simulink model "ctrl_student_HIL"  (R2015a)
settings: Solver=ode3  StartTime=0.0  StopTime=inf  FixedStep=0.01  RelTol=1e-3
undefined symbols (not defined in the file): DesiredPath, Elipscenter_radi, eta_dot_ini, K, K1, K2, l1, l2, l3, LAW, lim, lim_2, m, mu, pd, T_initialDP, U_ref
libraries: simulink x1
(part 4 of 4)

== matlab function ctrl_student_HIL/ControllerAndParanetrization/Controller1/Controller/Controller/MATLAB Function ==
  data: u input; D output; v input; r input
function D = fcn(u,v,r)
%% Damping coefficients
% Comments at the end of the lines indicate the old values used.
X_u		= -0.6555;		X_v		= 0;
X_uu 	= 0.3545;		X_vv	= -2.443;
X_uuu 	= -3.787;		X_vvv	= 0;

Y_v		= -1.33; 			Y_r		= -7.250; % Y_r
Y_vv	= -2.776;			Y_rr	= -3.450; % Y_rr
Y_vvv	= -64.91;			Y_rrr	= 0;
						
Y_rv	= -0.805;			Y_vr	= -0.845; % Y_rv, Y_vr

N_v		= 0;				N_r		= -1.900; % N_r
N_vv	= -0.2088;			N_rr	= -0.750; % N_rr
N_vvv	= 0;				N_rrr	= 0;
N_rv	= 0.130;			N_vr	= 0.080; % N_rv, N_vr
d_11 = -X_u - X_uu*u - X_uuu*u^2;
d_22 = -Y_v - Y_vv*v - Y_vvv*v^2 - Y_rv*abs(r);
d_33 = -N_r - N_rr*abs(r) - N_rrr*r^2 - N_vr*abs(v); % using abs(r)

d_12 = -X_v - X_vv*v - X_vvv*v^2;
d_23 = -Y_r - Y_rr*abs(r) - Y_rrr*r^2 - Y_vr*abs(v);
d_32 = -N_v - N_vv*v - N_vvv*v^2 - N_rv*abs(r);

D    = [d_11 0    0
        0    d_22 d_23
        0    d_32 d_33];
end

== matlab function ctrl_student_HIL/ControllerAndParanetrization/Controller1/Controller/Controller/MATLAB Function1 ==
  data: m input; M output
function M = fcn(m)
%% MATRICES

   I_z  =  1.7600;   x_g = 0.0375;       % x_g  =  0.0460; % Table B.1


%% Added mass
X_ud  =     -2.0;											% Table B.1
					Y_vd =     -1.0;	N_vd =    -0.0;		% Table B.1 guestimate
					Y_rd =      -0.0;	N_rd =    -1.0;		% Table B.1

%% Total mass matrix
m_11 = m-X_ud;
m_22 = m-Y_vd;
m_23 = m*x_g-Y_rd;
m_32 = m*x_g-N_vd;
m_33 = I_z-N_rd;

M    = [m_11 0    0
        0    m_22 m_23
        0    m_32 m_33];
end

== matlab function ctrl_student_HIL/ControllerAndParanetrization/Controller1/Controller/Controller/alpha_1dott/MATLAB Function ==
  data: K_1 input; alpha_1dott output; nu input; r input; eta_ds input; R_T input; U_s input; s_dot input; eta_dss input; U_ss input; z_1 input
function alpha_1dott = fcn(K_1,nu,r,eta_ds,R_T,U_s,s_dot,eta_dss,U_ss,z_1)
%% term 1
S_T=[0 r 0;-r 0 0;0 0 0];

term1=S_T*R_T*eta_ds*U_s;
%% term 2

term2=K_1*(-S_T*z_1-nu);
%% term 3

term3=K_1*R_T*eta_ds*s_dot;
%% term 4

term4=R_T*eta_dss*s_dot*U_s;
%% term 5 

term5=R_T*eta_ds*U_ss*s_dot;
%% summary

alpha_1dott=term1+term2+term3+term4+term5;
end

== matlab function ctrl_student_HIL/ThrustAllocationAndSaturation/actForces1 ==
  data: actSig input; tauAct output; satForces input
function tauAct  = act2Force(actSig,satForces)

t11=actSig(1)*satForces(1)*cos(actSig(3));
t12=actSig(2)*satForces(1)*cos(actSig(4));
t21=actSig(1)*satForces(1)*sin(actSig(3));
t22=actSig(2)*satForces(1)*sin(actSig(4));
t3=(t11-t12)*0.062-(t21+t22)*0.4575;

tauAct=[t11+t12;t21+t22;t3];

== matlab function ctrl_student_HIL/physics_model/kinetics ==
  data: tau input; nu_dot output; nu input
function nu_dot = CSE1_nu_dot_corr(tau,nu)

u   = nu(1);
v   = nu(2);
r   = nu(3);

tau = [tau(1);tau(2);tau(3)];
%% MATRICES

m    = 24.79;   I_z  =  1.7600;   x_g = 0.0375;       % x_g  =  0.0460; % Table B.1


%% Added mass
X_ud  =     -2.0;											% Table B.1
Y_vd =     -10.0;	
N_vd =    -0.0;                                             % Table B.1 guestimate
Y_rd =      -0.0;	
N_rd =    -1.0;                                             % Table B.1

%% Total mass matrix
m_11 = m-X_ud;
m_22 = m-Y_vd;
m_23 = m*x_g-Y_rd;
m_32 = m*x_g-N_vd;
m_33 = I_z-N_rd;

M    = [m_11 0    0
        0    m_22 m_23
        0    m_32 m_33];
	
%% Damping coefficients
% Comments at the end of the lines indicate the old values used.
X_u		= -0.6555;		X_v		= 0;
X_uu 	= 0.3545;		X_vv	= -2.443;
X_uuu 	= -3.787;		X_vvv	= 0;

Y_v		= -1.33; 			Y_r		= -7.250; % Y_r
Y_vv	= -2.776;			Y_rr	= -3.450; % Y_rr
Y_vvv	= -64.91;			Y_rrr	= 0;
						
Y_rv	= -0.805;			Y_vr	= -0.845; % Y_rv, Y_vr

N_v		= 0;				N_r		= -1.900; % N_r
N_vv	= -0.2088;			N_rr	= -0.750; % N_rr
N_vvv	= 0;				N_rrr	= 0;
N_rv	= 0.130;			N_vr	= 0.080; % N_rv, N_vr

%% Correolis matrix

%from ItsLearning
% c_13 = -(m-Y_vd)*v-(m*x_g-Y_rd)*r;
% c_23 = (m-X_ud)*u;
% C    = [0     0     c_13
%         0     0     c_23
%         -c_13 -c_23 0   ];

%From Handbook of Marine Craft Hydr 1st ed pp.120
a1 = X_ud*u;
a2 = Y_vd*v-m*x_g*r;
C    = [0     0     a2
        0     0    -a1
       -a2    a1    0   ];

%% Assembly of the damping matrix
d_11 = -X_u - X_uu*u - X_uuu*u^2;
d_22 = -Y_v - Y_vv*v - Y_vvv*v^2 - Y_rv*abs(r);
d_33 = -N_r - N_rr*abs(r) - N_rrr*r^2 - N_vr*abs(v); % using abs(r)

d_12 = -X_v - X_vv*v - X_vvv*v^2;
d_23 = -Y_r - Y_rr*abs(r) - Y_rrr*r^2 - Y_vr*abs(v);
d_32 = -N_v - N_vv*v - N_vvv*v^2 - N_rv*abs(r);

%From ItsLearning
% D    = [d_11 d_12 0
%         0    d_22 d_23
%         0    d_32 d_33];

%From Feb. 2017 lab manual. Agrees with Handbook of Marine Craft Hydro
D    = [d_11 0    0
        0    d_22 d_23
        0    d_32 d_33];



%% CALCULATION

%nu_dot = M\(tau-(C+D)*nu);
nu_dot = M\(tau-(D)*nu);

== matlab function ctrl_student_HIL/safety zone /MATLAB Function1 ==
  data: R input; R_T output
function R_T = fcn(R)
R_T=transpose(R);
end

== matlab function ctrl_student_HIL/ControllerAndParanetrization/Controller1/Control parameterization/BacksteppingParameterization /V_1s/Rotation Matrix ==
  data: yaw input; R output
function R = fcn(yaw)

R=[cos(yaw) -sin(yaw) 0;
    sin(yaw) cos(yaw) 0;
    0 0 1];

end

== matlab function ctrl_student_HIL/ControllerAndParanetrization/Controller1/Control parameterization/BacksteppingParameterization /Z_1/R Transposed ==
  data: R input; R_T output
function R_T = fcn(R)

R_T=transpose(R);

end

== matlab function ctrl_student_HIL/ControllerAndParanetrization/Controller1/Control parameterization/BacksteppingParameterization /Z_1/Rotation Matrix ==
  data: yaw input; R output
function R = fcn(yaw)

R=[cos(yaw) -sin(yaw) 0;
    sin(yaw) cos(yaw) 0;
    0 0 1];

end

== matlab function ctrl_student_HIL/ControllerAndParanetrization/PathParameterization/PathGenerization_Ellips/Check_s/CheckS&getU ==
  data: s_inn input; s_out output; U output; U_ref input; Switch output
function [s_out,U,Switch]= fcn(s_inn,U_ref)

if s_inn>=1
    s_out=0;
    Switch=0;
else
    s_out=s_inn;
    Switch=1;
end

U=U_ref/2;%U scaled again for the ellipsoidal case

end

== matlab function ctrl_student_HIL/ControllerAndParanetrization/PathParameterization/PathGenerization_Straight/Path parametization /Eta_ds/MATLAB Function ==
  data: x_d input; eta_ds_yaw output; y_d input; x_dd input; y_dd input
function eta_ds_yaw = fcn(x_d,y_d,x_dd,y_dd)

eta_ds_yaw=(x_d*y_dd-y_d*x_dd)/(y_d^2+x_d^2);

end

== matlab function ctrl_student_HIL/ControllerAndParanetrization/PathParameterization/PathGenerization_Straight/Path parametization /Eta_ds/MATLAB Function1 ==
  data: x_d input; x_dd output; y_d input; s input; y_dd output; x_dPrev input; y_dPrev input; s_Prev input; s1 output
function [x_dd,y_dd,s1]= fcn(x_d,y_d,s,x_dPrev,y_dPrev,s_Prev)

Delta_x=x_d-x_dPrev;
Delta_y=y_d-y_dPrev;
Delta_s=s-s_Prev;


x_dd=Delta_x/Delta_s;
y_dd=Delta_y/Delta_s;

s1=s;

end

== matlab function ctrl_student_HIL/ControllerAndParanetrization/PathParameterization/PathGenerization_Ellips/Path parametization /Subsystem/MATLAB Function ==
  data: Elipscenter_radi input; pd output; s input; pd_s output; eta_ds output; eta_dss output; U_ref input; U_ss output
function [pd,pd_s,eta_ds,eta_dss,U_ss] = fcn(Elipscenter_radi,s,U_ref)
pd=zeros(2,1);
pd_s=pd;
eta_ds=zeros(3,1);
eta_dss=zeros(3,1);

pd(1)=Elipscenter_radi(1,1)+cos(2*pi*s)*Elipscenter_radi(1,2);
pd(2)=Elipscenter_radi(2,1)+sin(2*pi*s)*Elipscenter_radi(2,2);

pd_s(1)=-2*pi*Elipscenter_radi(1,2)*sin(2*pi*s);
pd_s(2)=2*pi*Elipscenter_radi(2,2)*cos(2*pi*s);

eta_ds(1)=pd_s(1);
eta_ds(2)=pd_s(2);
x_dss=-4*pi^2*Elipscenter_radi(1,2)*cos(2*pi*s);
y_dss=-4*pi^2*Elipscenter_radi(2,2)*sin(2*pi*s);
x_ds=pd_s(1);
y_ds=pd_s(2);
eta_ds(3)=(x_ds*y_dss-x_dss*y_ds)/(x_ds^2+y_ds^2);
eta_dss(1)=x_dss;
eta_dss(2)=y_dss;

x_dsss=8*pi^3*Elipscenter_radi(1,2)*sin(2*pi*s);
y_dsss=-8*pi^3*Elipscenter_radi(2,2)*cos(2*pi*s);
term1=(x_ds*y_dsss-y_ds*x_dsss)/(x_ds^2+y_ds^2);
term2=-((x_ds*y_dss-y_ds*x_dss)*(2*x_ds*x_dss+2*y_ds*y_dss))/(x_ds^2+y_ds^2)^2;
eta_dss(3)=term1+term2;
U_ss=U_ref*(-x_ds*x_dss-y_ds*y_dss)/((x_ds^2+y_ds^2)^(1.5));
end

== matlab function ctrl_student_HIL/ControllerAndParanetrization/PathParameterization/PathGenerization_Ellips/parameter generator/MATLAB Function1 ==
  data: SwitchSignal_In input; SwitchSignal_Out output
function SwitchSignal_Out = fcn(SwitchSignal_In)

if SwitchSignal_In==0
    SwitchSignal_Out=1;
else
    SwitchSignal_Out=0;
end
    
end

== matlab function ctrl_student_HIL/ControllerAndParanetrization/PathParameterization/PathGenerization_Ellips/parameter generator/UpdateLaw ==
  data: s_dot output; p_d_sdot input; U_ref input; U_s output; V_1s input; mu input; eta_ds input; LAW input
function [s_dot,U_s ]= fcn(p_d_sdot,U_ref,V_1s,mu,eta_ds,LAW)


U_s=U_ref/(sqrt(p_d_sdot(1)^2+p_d_sdot(2)^2));
if LAW ==1

        s_dot=U_s-mu*V_1s;
else
        s_dot=U_s-mu/(sqrt(eta_ds(1)^2+eta_ds(2)^2))*V_1s;
end


end

== matlab function ctrl_student_HIL/ControllerAndParanetrization/PathParameterization/PathGenerization_Straight/Path parametization /Subsystem/MATLAB Function ==
  data: InitPosOut output; DesPos input; s_in input; U_ref input; N_iteration input; N_in input; DesPosOut output; SwitchSignal_out output; N_out output; U output; s_out output; Start_time input; init_time output; flag output
function [InitPosOut,DesPosOut,SwitchSignal_out,N_out,U,s_out,init_time,flag]= fcn(DesPos,s_in,U_ref,N_iteration,N_in,Start_time)
[a,b]=size(DesPos);
N_max=b-1;
    init_time=zeros(2,1);
    init_time(1)=Start_time(1)+1;
    init_time(2)=Start_time(2);
   

    
    
if init_time(1)<N_iteration         % DP for N_iterations
    N_out=N_in;
    InitPosOut=DesPos(:,N_out);
    DesPosOut=DesPos(:,N_out+1);
    SwitchSignal_out=1;
    s_out=0;
    DP=1;
    flag=1;
    
else
    if N_in==N_max                  % if we are at final stretch
        if  s_in>=0.9999
            N_out=N_in;
            InitPosOut=DesPos(:,N_out);
            DesPosOut=DesPos(:,N_out+1);
            SwitchSignal_out=1;
            s_out=1;
            DP=1;
            flag=2;
            
        else
            N_out=N_in;
            InitPosOut=DesPos(:,N_in);
            DesPosOut=DesPos(:,N_in+1);
            SwitchSignal_out=1;
            s_out=s_in;
            DP=0;
            flag=3;
            
        end
    else
       if s_in>=0.9999
           if N_in+1 ==N_max
               SwitchSignal_out=0;
               flag=40;
           else
               SwitchSignal_out=0;
               flag=50;
           end
            N_out=N_in+1;
            InitPosOut=DesPos(:,N_out);
            DesPosOut=DesPos(:,N_out+1);
            s_out=1;
            DP=0;

       else 
            if init_time(2)==0;
                init_time(2)=1;
                SwitchSignal_out=0;
                flag=5.75;
            else
                SwitchSignal_out=1;
                flag=5.25;
            end
            N_out=N_in;
            InitPosOut=DesPos(:,N_in);
            DesPosOut=DesPos(:,N_in+1);
            s_out=s_in;
            DP=0;
            
        end
    end
    
end   
if DP==1
    U=0;
else
    U=U_ref*(1.01+ sin(2*pi*s_out-pi/2));
end

end

== matlab function ctrl_student_HIL/ControllerAndParanetrization/PathParameterization/PathGenerization_Straight/parameter generator/MATLAB Function1 ==
  data: SwitchSignal_In input; SwitchSignal_Out output
function SwitchSignal_Out = fcn(SwitchSignal_In)

if SwitchSignal_In==0
    SwitchSignal_Out=1;
else
    SwitchSignal_Out=0;
end
    
end

== matlab function ctrl_student_HIL/ControllerAndParanetrization/PathParameterization/PathGenerization_Straight/parameter generator/UpdateLaw ==
  data: s_dot output; p_d_sdot input; U_ref input; U_s output; V_1s input; mu input; eta_ds input; LAW input
function [s_dot,U_s ]= fcn(p_d_sdot,U_ref,V_1s,mu,eta_ds,LAW)


U_s=U_ref/(sqrt(p_d_sdot(1)^2+p_d_sdot(2)^2));
if LAW ==1

        s_dot=U_s-mu*V_1s;
else
        s_dot=U_s-mu/(sqrt(eta_ds(1)^2+eta_ds(2)^2))*V_1s;
end


end

== matlab function ctrl_student_HIL/DPObserver1/Bias/bHatDot ==
  data: bHatDot output; L3 input; eta input; etaHat input
function bHatDot = fcn(L3,eta,etaHat)

bHatDot=L3*(eta-etaHat);
%bHatDot=[0;0;0];

end

== matlab function ctrl_student_HIL/DPObserver1/D ==
  data: D output; etaHatDot input
function D = fcn(etaHatDot)

u=etaHatDot(1);     %u=0; 
v=etaHatDot(2);     %v=0; 
r=etaHatDot(3);     %r=0;

Xu=-0.6555;
Xuu=0.3545;
Xuuu=-3.787;
Yv=-1.33;
Yvv=-2.776;
Yvvv=-64.91;
Yr=-7.25;
Yrr=-3.45;
Yrrr=0;
Yrv=-0.805;
Yvr=-0.845;
Nv=0;
Nvv=-0.2088;
Nvvv=0;
Nr=-1.9;
Nrr=-0.75;
Nrrr=0;
Nrv=0.13;
Nvr=0.08;

d11=-Xu-Xuu*abs(u)-Xuuu*u^2;
d22=-Yv-Yvv*abs(v)-Yvvv*v^2-Yrv*abs(r);
d23=-Yr-Yvr*abs(v)-Yrr*abs(r)-Yrrr*r^2;
d32=-Nv-Nvv*abs(v)-Nvvv*v^2-Nrv*abs(r);
d33=-Nr-Nvr*abs(v)-Nrr*abs(r)-Nrrr*r^2;

D=[d11 0 0; 0 d22 d23; 0 d32 d33];

end

== matlab function ctrl_student_HIL/DPObserver1/Subsystem/M ==
  data: M output
function M = void

m=14.79;
M=[m+2 0 0; 0 m+10 m*0.0375; 0 m*0.0375 1.76+1];

end

== matlab function ctrl_student_HIL/DPObserver1/Subsystem/nuHatDot ==
  data: nuHat input; bHat input; D input; M input; L2 input; tau input; eta input; R input; etaHat input; nuHatDot output
function nuHatDot = fcn(nuHat,bHat,D,M,L2,tau,eta,R,etaHat)

%nuHatDot=inv(M)*(-D*nuHat+transpose(R)*bHat+tau+K2*transpose(R)*L2*(eta-etaHat));

nuHatDot=inv(M)*(-D*nuHat+transpose(R)*bHat+tau+transpose(R)*L2*(eta-etaHat));

end

== matlab function ctrl_student_HIL/DPObserver1/calcR(psi)  ==
  data: psi input; R output
function R = fcn(psi)

R=[cos(psi) -sin(psi) 0; sin(psi) cos(psi) 0; 0 0 1];

end

== matlab function ctrl_student_HIL/DPObserver1/etaHat/etaHatDot ==
  data: etaHat input; nuHat input; L1 input; eta input; R input; etaHatDot output
function etaHatDot = fcn(etaHat,nuHat,L1,eta,R)

%etaHatDot=zeros(3,1);
etaHatDot=R*nuHat+L1*(eta-etaHat);

end
